simulink model "Transfer_Fcn_verif"  (Simulink 7.2)
settings: Solver=ode45  StartTime=0.0  StopTime=10.0  RelTol=1e-3
undefined symbols (not defined in the file): sample
settings Model: Creator=Romain  LastModifiedBy=Romain
settings OptimizationCC: ExpressionDepthLimit=128
settings DebuggingCC: SolverPrmCheckMsg=none  FcnCallInpInsideContextMsg=Enable All  StateNameClashWarn=none  StrictBusMsg=ErrorLevel1
settings CodeAppCC: CustomSymbolStrType=$N$R$M_T
settings GRTTargetCC: TargetFunctionLibrary=C89/C90 (ANSI)

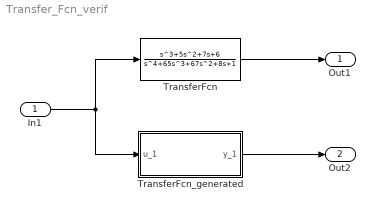
== system Transfer_Fcn_verif ==
  In1 : Inport  OutDataTypeStr=double  DataType=double
  TransferFcn : TransferFcn  Numerator=[1 5 7 6]  Denominator=[1 65 67 8 1]
  TransferFcn_generated : Subsystem  TreatAsAtomicUnit=on
  Out1 : Outport
  Out2 : Outport  Port=2
  wires:
  In1/1 -> TransferFcn_generated/1(u_1), TransferFcn/1
  TransferFcn/1 -> Out1/1
  TransferFcn_generated/1(y_1) -> Out2/1

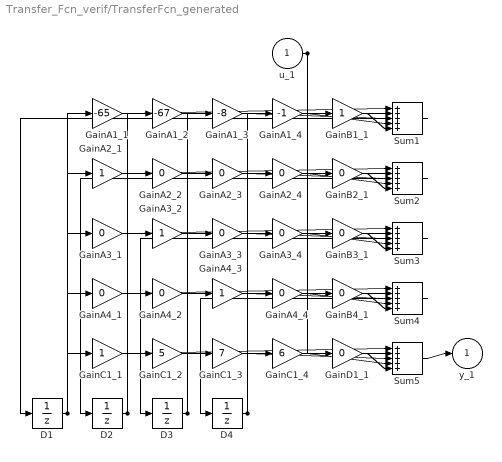
== system Transfer_Fcn_verif/TransferFcn_generated ==
  u_1 : Inport
  D{1..4} (4 alike) : UnitDelay  SampleTime=sample
  GainA1_1 : Gain  Gain=-65  SaturateOnIntegerOverflow=on  OutDataTypeStr=Inherit: Same as input  ParamDataTypeStr=Inherit: Same as input
  GainA1_2 : Gain  Gain=-67  SaturateOnIntegerOverflow=on  OutDataTypeStr=Inherit: Same as input  ParamDataTypeStr=Inherit: Same as input
  GainA1_3 : Gain  Gain=-8  SaturateOnIntegerOverflow=on  OutDataTypeStr=Inherit: Same as input  ParamDataTypeStr=Inherit: Same as input
  GainA1_4 : Gain  Gain=-1  SaturateOnIntegerOverflow=on  OutDataTypeStr=Inherit: Same as input  ParamDataTypeStr=Inherit: Same as input
  GainA2_1 : Gain  SaturateOnIntegerOverflow=on  OutDataTypeStr=Inherit: Same as input  ParamDataTypeStr=Inherit: Same as input
  GainA2_2 : Gain  Gain=0  SaturateOnIntegerOverflow=on  OutDataTypeStr=Inherit: Same as input  ParamDataTypeStr=Inherit: Same as input
  GainA2_3 : Gain  Gain=0  SaturateOnIntegerOverflow=on  OutDataTypeStr=Inherit: Same as input  ParamDataTypeStr=Inherit: Same as input
  GainA2_4 : Gain  Gain=0  SaturateOnIntegerOverflow=on  OutDataTypeStr=Inherit: Same as input  ParamDataTypeStr=Inherit: Same as input
  GainA3_1 : Gain  Gain=0  SaturateOnIntegerOverflow=on  OutDataTypeStr=Inherit: Same as input  ParamDataTypeStr=Inherit: Same as input
  GainA3_2 : Gain  SaturateOnIntegerOverflow=on  OutDataTypeStr=Inherit: Same as input  ParamDataTypeStr=Inherit: Same as input
  GainA3_3 : Gain  Gain=0  SaturateOnIntegerOverflow=on  OutDataTypeStr=Inherit: Same as input  ParamDataTypeStr=Inherit: Same as input
  GainA3_4 : Gain  Gain=0  SaturateOnIntegerOverflow=on  OutDataTypeStr=Inherit: Same as input  ParamDataTypeStr=Inherit: Same as input
  GainA4_1 : Gain  Gain=0  SaturateOnIntegerOverflow=on  OutDataTypeStr=Inherit: Same as input  ParamDataTypeStr=Inherit: Same as input
  GainA4_2 : Gain  Gain=0  SaturateOnIntegerOverflow=on  OutDataTypeStr=Inherit: Same as input  ParamDataTypeStr=Inherit: Same as input
  GainA4_3 : Gain  SaturateOnIntegerOverflow=on  OutDataTypeStr=Inherit: Same as input  ParamDataTypeStr=Inherit: Same as input
  GainA4_4 : Gain  Gain=0  SaturateOnIntegerOverflow=on  OutDataTypeStr=Inherit: Same as input  ParamDataTypeStr=Inherit: Same as input
  GainB1_1 : Gain  SaturateOnIntegerOverflow=on  OutDataTypeStr=Inherit: Same as input  ParamDataTypeStr=Inherit: Same as input
  GainB2_1 : Gain  Gain=0  SaturateOnIntegerOverflow=on  OutDataTypeStr=Inherit: Same as input  ParamDataTypeStr=Inherit: Same as input
  GainB3_1 : Gain  Gain=0  SaturateOnIntegerOverflow=on  OutDataTypeStr=Inherit: Same as input  ParamDataTypeStr=Inherit: Same as input
  GainB4_1 : Gain  Gain=0  SaturateOnIntegerOverflow=on  OutDataTypeStr=Inherit: Same as input  ParamDataTypeStr=Inherit: Same as input
  GainC1_1 : Gain  SaturateOnIntegerOverflow=on  OutDataTypeStr=Inherit: Same as input  ParamDataTypeStr=Inherit: Same as input
  GainC1_2 : Gain  Gain=5  SaturateOnIntegerOverflow=on  OutDataTypeStr=Inherit: Same as input  ParamDataTypeStr=Inherit: Same as input
  GainC1_3 : Gain  Gain=7  SaturateOnIntegerOverflow=on  OutDataTypeStr=Inherit: Same as input  ParamDataTypeStr=Inherit: Same as input
  GainC1_4 : Gain  Gain=6  SaturateOnIntegerOverflow=on  OutDataTypeStr=Inherit: Same as input  ParamDataTypeStr=Inherit: Same as input
  GainD1_1 : Gain  Gain=0  SaturateOnIntegerOverflow=on  OutDataTypeStr=Inherit: Same as input  ParamDataTypeStr=Inherit: Same as input
  Sum{1..5} (5 alike) : Sum  Inputs=+++++  SaturateOnIntegerOverflow=on  InputSameDT=on  OutDataTypeStr=Inherit: Same as first input
  y_1 : Outport
  wires:
  D1/1 -> GainA1_1/1, GainA2_1/1, GainA3_1/1, GainA4_1/1, GainC1_1/1
  GainA1_1/1 -> Sum1/1
  D2/1 -> GainA1_2/1, GainA2_2/1, GainA3_2/1, GainA4_2/1, GainC1_2/1
  GainA1_2/1 -> Sum1/2
  D3/1 -> GainA1_3/1, GainA2_3/1, GainA3_3/1, GainA4_3/1, GainC1_3/1
  GainA1_3/1 -> Sum1/3
  D4/1 -> GainA1_4/1, GainA2_4/1, GainA3_4/1, GainA4_4/1, GainC1_4/1
  GainA1_4/1 -> Sum1/4
  GainA2_1/1 -> Sum2/1
  GainA2_2/1 -> Sum2/2
  GainA2_3/1 -> Sum2/3
  GainA2_4/1 -> Sum2/4
  GainA3_1/1 -> Sum3/1
  GainA3_2/1 -> Sum3/2
  GainA3_3/1 -> Sum3/3
  GainA3_4/1 -> Sum3/4
  GainA4_1/1 -> Sum4/1
  GainA4_2/1 -> Sum4/2
  GainA4_3/1 -> Sum4/3
  GainA4_4/1 -> Sum4/4
  GainC1_1/1 -> Sum5/1
  GainC1_2/1 -> Sum5/2
  GainC1_3/1 -> Sum5/3
  GainC1_4/1 -> Sum5/4
  u_1/1 -> GainB1_1/1, GainB2_1/1, GainB3_1/1, GainB4_1/1, GainD1_1/1
  GainB1_1/1 -> Sum1/5
  GainB2_1/1 -> Sum2/5
  GainB3_1/1 -> Sum3/5
  GainB4_1/1 -> Sum4/5
  GainD1_1/1 -> Sum5/5
  Sum1/1 -> D1/1
  Sum2/1 -> D2/1
  Sum3/1 -> D3/1
  Sum4/1 -> D4/1
  Sum5/1 -> y_1/1
